simulink model "MATE_9LevelDrive_LowHarmonicRectifier"  (R2024b)
settings: Solver=FixedStepDiscrete  StartTime=0.0  StopTime=1  FixedStep=Ts  RelTol=1e-3
PostLoadFcn:
  | Ts=25e-6; initDrive9Level;Rsnu=30; Csnu=3e-6;Ron=0.01;Roff=1e6; Vf=2;
InitFcn:
  | Ts=25e-6; initDrive9Level;Rsnu=30; Csnu=3e-6;Ron=0.01;Roff=1e6; Vf=2;
values from neighbouring files (symbols this model uses):
  Lbase = Zbase/wbase    (= 0.0044902914611)    [initDrive9Level.m]
  Rgnd_rectifier = 1e4    (= 10000)    [initDrive9Level.m]
  T_2wind_ratio = 0.2677    [initDrive9Level.m]
  T_Lpu = Ltot_pu*9/10    (= 0.036)    [initDrive9Level.m]
  T_Lpu_pri = Ltot_pu/10    (= 0.004)    [initDrive9Level.m]
  T_Rpu = Rtot_pu*9/10    (= 0.009)    [initDrive9Level.m]
  T_Rpu_pri = Rtot_pu/10    (= 0.001)    [initDrive9Level.m]
  T_Vpri = 3000    [initDrive9Level.m]
  T_Vpri_15comp = 1.1168    [initDrive9Level.m]
  T_Vsec = 920    [initDrive9Level.m]
  Zbase = T_Vsec*T_Vsec/T_Pbase    (= 1.6928)    [initDrive9Level.m]
undefined symbols (not defined in the file or in its folder): DiscIntNeverNeededParam, gcbh, sps_rtmsupport
libraries: fl_lib x192, ee_lib x105, simetranss x26, nesl_utility x21
(part 5 of 5)

== system MATE_9LevelDrive_LowHarmonicRectifier/ModulationSimulink/Signal out ==
  freq(Hz) : Inport
  x : Inport  Port=2
  1pu-> 4 DC stage : Gain  Gain=4  SaturateOnIntegerOverflow=on  OutDataTypeStr=Inherit: Same as input  ParamDataTypeStr=Inherit: Same as input
  2*pi1 : Gain  Gain=2*pi  SaturateOnIntegerOverflow=on  OutDataTypeStr=Inherit: Same as input  ParamDataTypeStr=Inherit: Same as input
  Discrete-Time Integrator2 : DiscreteIntegrator  SampleTime=Ts  ICPrevOutput=DiscIntNeverNeededParam  ICPrevScaledInput=DiscIntNeverNeededParam
  Product : Product  SaturateOnIntegerOverflow=on  OutDataTypeStr=Inherit: Same as first input
  Sum : Sum  Inputs=|++  SaturateOnIntegerOverflow=on
  Trigonometric Function3 : Trigonometry
  phase : Constant  Value=[0 2*pi/3 -2*pi/3]
  Out1 : Outport  VectorParamsAs1DForOutWhenUnconnected=off
  wires:
  x/1 -> 1pu-> 4 DC stage/1
  Product/1 -> Out1/1
  1pu-> 4 DC stage/1 -> Product/2
  Trigonometric Function3/1 -> Product/1
  freq(Hz)/1 -> 2*pi1/1
  phase/1 -> Sum/2
  Sum/1 -> Trigonometric Function3/1
  Discrete-Time Integrator2/1 -> Sum/1
  2*pi1/1 -> Discrete-Time Integrator2/1

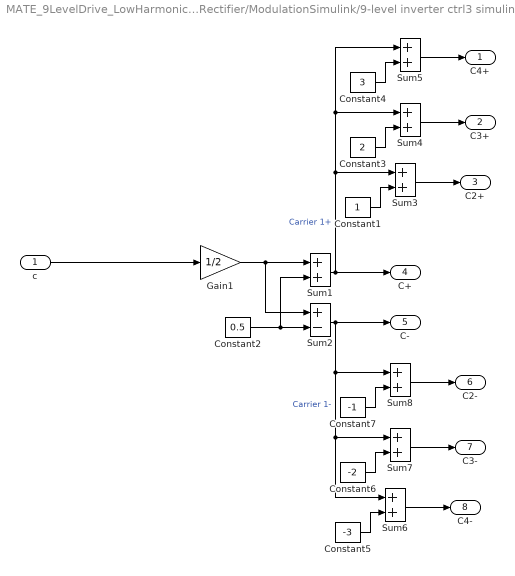
== system MATE_9LevelDrive_LowHarmonicRectifier/ModulationSimulink/9-level inverter ctrl3 simulink/Carriers Generator ==
  c : Inport
  Constant1 : Constant
  Constant2 : Constant  Value=0.5
  Constant3 : Constant  Value=2
  Constant4 : Constant  Value=3
  Constant5 : Constant  Value=-3
  Constant6 : Constant  Value=-2
  Constant7 : Constant  Value=-1
  Gain1 : Gain  Gain=1/2  SaturateOnIntegerOverflow=on  OutDataTypeStr=Inherit: Same as input  ParamDataTypeStr=Inherit: Same as input
  Sum{1,3..8} (7 alike) : Sum  InputSameDT=on  SaturateOnIntegerOverflow=on  OutDataTypeStr=Inherit: Same as first input
  Sum2 : Sum  Inputs=+-  InputSameDT=on  SaturateOnIntegerOverflow=on  OutDataTypeStr=Inherit: Same as first input
  C4+ : Outport  VectorParamsAs1DForOutWhenUnconnected=off
  C3+ : Outport  Port=2  VectorParamsAs1DForOutWhenUnconnected=off
  C2+ : Outport  Port=3  VectorParamsAs1DForOutWhenUnconnected=off
  C+ : Outport  Port=4  VectorParamsAs1DForOutWhenUnconnected=off
  C- : Outport  Port=5  VectorParamsAs1DForOutWhenUnconnected=off
  C2- : Outport  Port=6  VectorParamsAs1DForOutWhenUnconnected=off
  C3- : Outport  Port=7  VectorParamsAs1DForOutWhenUnconnected=off
  C4- : Outport  Port=8  VectorParamsAs1DForOutWhenUnconnected=off
  wires:
  c/1 -> Gain1/1
  Sum1/1 -> C+/1, Sum3/1, Sum4/1, Sum5/1  "Carrier 1+"
  Sum2/1 -> C-/1, Sum8/1, Sum7/1, Sum6/1  "Carrier 1-"
  Constant2/1 -> Sum1/2, Sum2/2
  Gain1/1 -> Sum2/1, Sum1/1
  Sum3/1 -> C2+/1
  Constant1/1 -> Sum3/2
  Sum4/1 -> C3+/1
  Constant3/1 -> Sum4/2
  Sum5/1 -> C4+/1
  Constant4/1 -> Sum5/2
  Sum6/1 -> C4-/1
  Constant5/1 -> Sum6/2
  Sum7/1 -> C3-/1
  Constant6/1 -> Sum7/2
  Sum8/1 -> C2-/1
  Constant7/1 -> Sum8/2

== system MATE_9LevelDrive_LowHarmonicRectifier/ModulationSimulink/9-level inverter ctrl3 simulink/rte1 ==
  in : Inport
  c+ : Inport  Port=2
  c- : Inport  Port=3
  Logical Operator : Logic  Operator=NOT  AllPortsSameDT=off  OutDataTypeStr=boolean
  Logical Operator1 : Logic  Operator=NOT  AllPortsSameDT=off  OutDataTypeStr=boolean
  Relational Operator : RelationalOperator  Operator=>  OutDataTypeStr=boolean  RndMeth=Simplest  InputSameDT=off
  Relational Operator1 : RelationalOperator  Operator=<  OutDataTypeStr=boolean  RndMeth=Simplest  InputSameDT=off
  1 : Outport  VectorParamsAs1DForOutWhenUnconnected=off
  2 : Outport  Port=2  VectorParamsAs1DForOutWhenUnconnected=off
  3 : Outport  Port=3  VectorParamsAs1DForOutWhenUnconnected=off
  4 : Outport  Port=4  VectorParamsAs1DForOutWhenUnconnected=off
  wires:
  Logical Operator1/1 -> 4/1
  Logical Operator/1 -> 2/1
  Relational Operator1/1 -> 3/1, Logical Operator1/1
  Relational Operator/1 -> 1/1, Logical Operator/1
  c-/1 -> Relational Operator1/2
  c+/1 -> Relational Operator/2
  in/1 -> Relational Operator/1, Relational Operator1/1

== system MATE_9LevelDrive_LowHarmonicRectifier/ModulationSimulink/9-level inverter ctrl3 simulink/rte2 ==
  in : Inport
  c+ : Inport  Port=2
  c- : Inport  Port=3
  Logical Operator : Logic  Operator=NOT  AllPortsSameDT=off  OutDataTypeStr=boolean
  Logical Operator1 : Logic  Operator=NOT  AllPortsSameDT=off  OutDataTypeStr=boolean
  Relational Operator : RelationalOperator  Operator=>  OutDataTypeStr=boolean  RndMeth=Simplest  InputSameDT=off
  Relational Operator1 : RelationalOperator  Operator=<  OutDataTypeStr=boolean  RndMeth=Simplest  InputSameDT=off
  1 : Outport  VectorParamsAs1DForOutWhenUnconnected=off
  2 : Outport  Port=2  VectorParamsAs1DForOutWhenUnconnected=off
  3 : Outport  Port=3  VectorParamsAs1DForOutWhenUnconnected=off
  4 : Outport  Port=4  VectorParamsAs1DForOutWhenUnconnected=off
  wires:
  in/1 -> Relational Operator1/1, Relational Operator/1
  c+/1 -> Relational Operator/2
  c-/1 -> Relational Operator1/2
  Relational Operator/1 -> Logical Operator/1, 1/1
  Relational Operator1/1 -> Logical Operator1/1, 3/1
  Logical Operator/1 -> 2/1
  Logical Operator1/1 -> 4/1

== system MATE_9LevelDrive_LowHarmonicRectifier/ModulationSimulink/9-level inverter ctrl3 simulink/rte3 ==
  in : Inport
  c+ : Inport  Port=2
  c- : Inport  Port=3
  Logical Operator : Logic  Operator=NOT  AllPortsSameDT=off  OutDataTypeStr=boolean
  Logical Operator1 : Logic  Operator=NOT  AllPortsSameDT=off  OutDataTypeStr=boolean
  Relational Operator : RelationalOperator  Operator=>  OutDataTypeStr=boolean  RndMeth=Simplest  InputSameDT=off
  Relational Operator1 : RelationalOperator  Operator=<  OutDataTypeStr=boolean  RndMeth=Simplest  InputSameDT=off
  1 : Outport  VectorParamsAs1DForOutWhenUnconnected=off
  2 : Outport  Port=2  VectorParamsAs1DForOutWhenUnconnected=off
  3 : Outport  Port=3  VectorParamsAs1DForOutWhenUnconnected=off
  4 : Outport  Port=4  VectorParamsAs1DForOutWhenUnconnected=off
  wires:
  in/1 -> Relational Operator1/1, Relational Operator/1
  c+/1 -> Relational Operator/2
  c-/1 -> Relational Operator1/2
  Relational Operator/1 -> Logical Operator/1, 1/1
  Relational Operator1/1 -> Logical Operator1/1, 3/1
  Logical Operator/1 -> 2/1
  Logical Operator1/1 -> 4/1

== system MATE_9LevelDrive_LowHarmonicRectifier/ModulationSimulink/9-level inverter ctrl3 simulink/rte4 ==
  in : Inport
  c+ : Inport  Port=2
  c- : Inport  Port=3
  Logical Operator : Logic  Operator=NOT  AllPortsSameDT=off  OutDataTypeStr=boolean
  Logical Operator1 : Logic  Operator=NOT  AllPortsSameDT=off  OutDataTypeStr=boolean
  Relational Operator : RelationalOperator  Operator=>  OutDataTypeStr=boolean  RndMeth=Simplest  InputSameDT=off
  Relational Operator1 : RelationalOperator  Operator=<  OutDataTypeStr=boolean  RndMeth=Simplest  InputSameDT=off
  1 : Outport  VectorParamsAs1DForOutWhenUnconnected=off
  2 : Outport  Port=2  VectorParamsAs1DForOutWhenUnconnected=off
  3 : Outport  Port=3  VectorParamsAs1DForOutWhenUnconnected=off
  4 : Outport  Port=4  VectorParamsAs1DForOutWhenUnconnected=off
  wires:
  Logical Operator1/1 -> 4/1
  Logical Operator/1 -> 2/1
  Relational Operator1/1 -> 3/1, Logical Operator1/1
  Relational Operator/1 -> 1/1, Logical Operator/1
  c-/1 -> Relational Operator1/2
  c+/1 -> Relational Operator/2
  in/1 -> Relational Operator/1, Relational Operator1/1

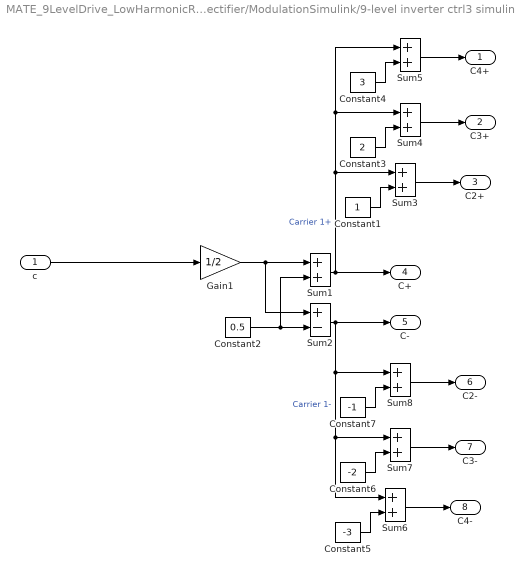
== system MATE_9LevelDrive_LowHarmonicRectifier/ModulationSimulink/9-level inverter ctrl3 simulink1/Carriers Generator ==
  c : Inport
  Constant1 : Constant
  Constant2 : Constant  Value=0.5
  Constant3 : Constant  Value=2
  Constant4 : Constant  Value=3
  Constant5 : Constant  Value=-3
  Constant6 : Constant  Value=-2
  Constant7 : Constant  Value=-1
  Gain1 : Gain  Gain=1/2  SaturateOnIntegerOverflow=on  OutDataTypeStr=Inherit: Same as input  ParamDataTypeStr=Inherit: Same as input
  Sum{1,3..8} (7 alike) : Sum  InputSameDT=on  SaturateOnIntegerOverflow=on  OutDataTypeStr=Inherit: Same as first input
  Sum2 : Sum  Inputs=+-  InputSameDT=on  SaturateOnIntegerOverflow=on  OutDataTypeStr=Inherit: Same as first input
  C4+ : Outport  VectorParamsAs1DForOutWhenUnconnected=off
  C3+ : Outport  Port=2  VectorParamsAs1DForOutWhenUnconnected=off
  C2+ : Outport  Port=3  VectorParamsAs1DForOutWhenUnconnected=off
  C+ : Outport  Port=4  VectorParamsAs1DForOutWhenUnconnected=off
  C- : Outport  Port=5  VectorParamsAs1DForOutWhenUnconnected=off
  C2- : Outport  Port=6  VectorParamsAs1DForOutWhenUnconnected=off
  C3- : Outport  Port=7  VectorParamsAs1DForOutWhenUnconnected=off
  C4- : Outport  Port=8  VectorParamsAs1DForOutWhenUnconnected=off
  wires:
  Constant7/1 -> Sum8/2
  Sum8/1 -> C2-/1
  Constant6/1 -> Sum7/2
  Sum7/1 -> C3-/1
  Constant5/1 -> Sum6/2
  Sum6/1 -> C4-/1
  Constant4/1 -> Sum5/2
  Sum5/1 -> C4+/1
  Constant3/1 -> Sum4/2
  Sum4/1 -> C3+/1
  Constant1/1 -> Sum3/2
  Sum3/1 -> C2+/1
  Gain1/1 -> Sum1/1, Sum2/1
  Constant2/1 -> Sum2/2, Sum1/2
  Sum2/1 -> Sum6/1, Sum7/1, Sum8/1, C-/1  "Carrier 1-"
  Sum1/1 -> Sum5/1, Sum4/1, Sum3/1, C+/1  "Carrier 1+"
  c/1 -> Gain1/1

== system MATE_9LevelDrive_LowHarmonicRectifier/ModulationSimulink/9-level inverter ctrl3 simulink1/rte1 ==
  in : Inport
  c+ : Inport  Port=2
  c- : Inport  Port=3
  Logical Operator : Logic  Operator=NOT  AllPortsSameDT=off  OutDataTypeStr=boolean
  Logical Operator1 : Logic  Operator=NOT  AllPortsSameDT=off  OutDataTypeStr=boolean
  Relational Operator : RelationalOperator  Operator=>  OutDataTypeStr=boolean  RndMeth=Simplest  InputSameDT=off
  Relational Operator1 : RelationalOperator  Operator=<  OutDataTypeStr=boolean  RndMeth=Simplest  InputSameDT=off
  1 : Outport  VectorParamsAs1DForOutWhenUnconnected=off
  2 : Outport  Port=2  VectorParamsAs1DForOutWhenUnconnected=off
  3 : Outport  Port=3  VectorParamsAs1DForOutWhenUnconnected=off
  4 : Outport  Port=4  VectorParamsAs1DForOutWhenUnconnected=off
  wires:
  in/1 -> Relational Operator1/1, Relational Operator/1
  c+/1 -> Relational Operator/2
  c-/1 -> Relational Operator1/2
  Relational Operator/1 -> Logical Operator/1, 1/1
  Relational Operator1/1 -> Logical Operator1/1, 3/1
  Logical Operator/1 -> 2/1
  Logical Operator1/1 -> 4/1

== system MATE_9LevelDrive_LowHarmonicRectifier/ModulationSimulink/9-level inverter ctrl3 simulink1/rte2 ==
  in : Inport
  c+ : Inport  Port=2
  c- : Inport  Port=3
  Logical Operator : Logic  Operator=NOT  AllPortsSameDT=off  OutDataTypeStr=boolean
  Logical Operator1 : Logic  Operator=NOT  AllPortsSameDT=off  OutDataTypeStr=boolean
  Relational Operator : RelationalOperator  Operator=>  OutDataTypeStr=boolean  RndMeth=Simplest  InputSameDT=off
  Relational Operator1 : RelationalOperator  Operator=<  OutDataTypeStr=boolean  RndMeth=Simplest  InputSameDT=off
  1 : Outport  VectorParamsAs1DForOutWhenUnconnected=off
  2 : Outport  Port=2  VectorParamsAs1DForOutWhenUnconnected=off
  3 : Outport  Port=3  VectorParamsAs1DForOutWhenUnconnected=off
  4 : Outport  Port=4  VectorParamsAs1DForOutWhenUnconnected=off
  wires:
  Logical Operator1/1 -> 4/1
  Logical Operator/1 -> 2/1
  Relational Operator1/1 -> 3/1, Logical Operator1/1
  Relational Operator/1 -> 1/1, Logical Operator/1
  c-/1 -> Relational Operator1/2
  c+/1 -> Relational Operator/2
  in/1 -> Relational Operator/1, Relational Operator1/1

== system MATE_9LevelDrive_LowHarmonicRectifier/ModulationSimulink/9-level inverter ctrl3 simulink1/rte3 ==
  in : Inport
  c+ : Inport  Port=2
  c- : Inport  Port=3
  Logical Operator : Logic  Operator=NOT  AllPortsSameDT=off  OutDataTypeStr=boolean
  Logical Operator1 : Logic  Operator=NOT  AllPortsSameDT=off  OutDataTypeStr=boolean
  Relational Operator : RelationalOperator  Operator=>  OutDataTypeStr=boolean  RndMeth=Simplest  InputSameDT=off
  Relational Operator1 : RelationalOperator  Operator=<  OutDataTypeStr=boolean  RndMeth=Simplest  InputSameDT=off
  1 : Outport  VectorParamsAs1DForOutWhenUnconnected=off
  2 : Outport  Port=2  VectorParamsAs1DForOutWhenUnconnected=off
  3 : Outport  Port=3  VectorParamsAs1DForOutWhenUnconnected=off
  4 : Outport  Port=4  VectorParamsAs1DForOutWhenUnconnected=off
  wires:
  Logical Operator1/1 -> 4/1
  Logical Operator/1 -> 2/1
  Relational Operator1/1 -> 3/1, Logical Operator1/1
  Relational Operator/1 -> 1/1, Logical Operator/1
  c-/1 -> Relational Operator1/2
  c+/1 -> Relational Operator/2
  in/1 -> Relational Operator/1, Relational Operator1/1

== system MATE_9LevelDrive_LowHarmonicRectifier/ModulationSimulink/9-level inverter ctrl3 simulink1/rte4 ==
  in : Inport
  c+ : Inport  Port=2
  c- : Inport  Port=3
  Logical Operator : Logic  Operator=NOT  AllPortsSameDT=off  OutDataTypeStr=boolean
  Logical Operator1 : Logic  Operator=NOT  AllPortsSameDT=off  OutDataTypeStr=boolean
  Relational Operator : RelationalOperator  Operator=>  OutDataTypeStr=boolean  RndMeth=Simplest  InputSameDT=off
  Relational Operator1 : RelationalOperator  Operator=<  OutDataTypeStr=boolean  RndMeth=Simplest  InputSameDT=off
  1 : Outport  VectorParamsAs1DForOutWhenUnconnected=off
  2 : Outport  Port=2  VectorParamsAs1DForOutWhenUnconnected=off
  3 : Outport  Port=3  VectorParamsAs1DForOutWhenUnconnected=off
  4 : Outport  Port=4  VectorParamsAs1DForOutWhenUnconnected=off
  wires:
  in/1 -> Relational Operator1/1, Relational Operator/1
  c+/1 -> Relational Operator/2
  c-/1 -> Relational Operator1/2
  Relational Operator/1 -> Logical Operator/1, 1/1
  Relational Operator1/1 -> Logical Operator1/1, 3/1
  Logical Operator/1 -> 2/1
  Logical Operator1/1 -> 4/1

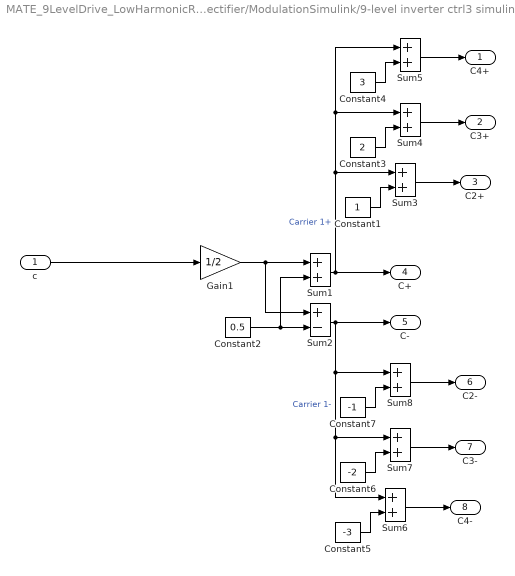
== system MATE_9LevelDrive_LowHarmonicRectifier/ModulationSimulink/9-level inverter ctrl3 simulink2/Carriers Generator ==
  c : Inport
  Constant1 : Constant
  Constant2 : Constant  Value=0.5
  Constant3 : Constant  Value=2
  Constant4 : Constant  Value=3
  Constant5 : Constant  Value=-3
  Constant6 : Constant  Value=-2
  Constant7 : Constant  Value=-1
  Gain1 : Gain  Gain=1/2  SaturateOnIntegerOverflow=on  OutDataTypeStr=Inherit: Same as input  ParamDataTypeStr=Inherit: Same as input
  Sum{1,3..8} (7 alike) : Sum  InputSameDT=on  SaturateOnIntegerOverflow=on  OutDataTypeStr=Inherit: Same as first input
  Sum2 : Sum  Inputs=+-  InputSameDT=on  SaturateOnIntegerOverflow=on  OutDataTypeStr=Inherit: Same as first input
  C4+ : Outport  VectorParamsAs1DForOutWhenUnconnected=off
  C3+ : Outport  Port=2  VectorParamsAs1DForOutWhenUnconnected=off
  C2+ : Outport  Port=3  VectorParamsAs1DForOutWhenUnconnected=off
  C+ : Outport  Port=4  VectorParamsAs1DForOutWhenUnconnected=off
  C- : Outport  Port=5  VectorParamsAs1DForOutWhenUnconnected=off
  C2- : Outport  Port=6  VectorParamsAs1DForOutWhenUnconnected=off
  C3- : Outport  Port=7  VectorParamsAs1DForOutWhenUnconnected=off
  C4- : Outport  Port=8  VectorParamsAs1DForOutWhenUnconnected=off
  wires:
  c/1 -> Gain1/1
  Sum1/1 -> C+/1, Sum3/1, Sum4/1, Sum5/1  "Carrier 1+"
  Sum2/1 -> C-/1, Sum8/1, Sum7/1, Sum6/1  "Carrier 1-"
  Constant2/1 -> Sum1/2, Sum2/2
  Gain1/1 -> Sum2/1, Sum1/1
  Sum3/1 -> C2+/1
  Constant1/1 -> Sum3/2
  Sum4/1 -> C3+/1
  Constant3/1 -> Sum4/2
  Sum5/1 -> C4+/1
  Constant4/1 -> Sum5/2
  Sum6/1 -> C4-/1
  Constant5/1 -> Sum6/2
  Sum7/1 -> C3-/1
  Constant6/1 -> Sum7/2
  Sum8/1 -> C2-/1
  Constant7/1 -> Sum8/2

== system MATE_9LevelDrive_LowHarmonicRectifier/ModulationSimulink/9-level inverter ctrl3 simulink2/rte1 ==
  in : Inport
  c+ : Inport  Port=2
  c- : Inport  Port=3
  Logical Operator : Logic  Operator=NOT  AllPortsSameDT=off  OutDataTypeStr=boolean
  Logical Operator1 : Logic  Operator=NOT  AllPortsSameDT=off  OutDataTypeStr=boolean
  Relational Operator : RelationalOperator  Operator=>  OutDataTypeStr=boolean  RndMeth=Simplest  InputSameDT=off
  Relational Operator1 : RelationalOperator  Operator=<  OutDataTypeStr=boolean  RndMeth=Simplest  InputSameDT=off
  1 : Outport  VectorParamsAs1DForOutWhenUnconnected=off
  2 : Outport  Port=2  VectorParamsAs1DForOutWhenUnconnected=off
  3 : Outport  Port=3  VectorParamsAs1DForOutWhenUnconnected=off
  4 : Outport  Port=4  VectorParamsAs1DForOutWhenUnconnected=off
  wires:
  Logical Operator1/1 -> 4/1
  Logical Operator/1 -> 2/1
  Relational Operator1/1 -> 3/1, Logical Operator1/1
  Relational Operator/1 -> 1/1, Logical Operator/1
  c-/1 -> Relational Operator1/2
  c+/1 -> Relational Operator/2
  in/1 -> Relational Operator/1, Relational Operator1/1

== system MATE_9LevelDrive_LowHarmonicRectifier/ModulationSimulink/9-level inverter ctrl3 simulink2/rte2 ==
  in : Inport
  c+ : Inport  Port=2
  c- : Inport  Port=3
  Logical Operator : Logic  Operator=NOT  AllPortsSameDT=off  OutDataTypeStr=boolean
  Logical Operator1 : Logic  Operator=NOT  AllPortsSameDT=off  OutDataTypeStr=boolean
  Relational Operator : RelationalOperator  Operator=>  OutDataTypeStr=boolean  RndMeth=Simplest  InputSameDT=off
  Relational Operator1 : RelationalOperator  Operator=<  OutDataTypeStr=boolean  RndMeth=Simplest  InputSameDT=off
  1 : Outport  VectorParamsAs1DForOutWhenUnconnected=off
  2 : Outport  Port=2  VectorParamsAs1DForOutWhenUnconnected=off
  3 : Outport  Port=3  VectorParamsAs1DForOutWhenUnconnected=off
  4 : Outport  Port=4  VectorParamsAs1DForOutWhenUnconnected=off
  wires:
  in/1 -> Relational Operator1/1, Relational Operator/1
  c+/1 -> Relational Operator/2
  c-/1 -> Relational Operator1/2
  Relational Operator/1 -> Logical Operator/1, 1/1
  Relational Operator1/1 -> Logical Operator1/1, 3/1
  Logical Operator/1 -> 2/1
  Logical Operator1/1 -> 4/1

== system MATE_9LevelDrive_LowHarmonicRectifier/ModulationSimulink/9-level inverter ctrl3 simulink2/rte3 ==
  in : Inport
  c+ : Inport  Port=2
  c- : Inport  Port=3
  Logical Operator : Logic  Operator=NOT  AllPortsSameDT=off  OutDataTypeStr=boolean
  Logical Operator1 : Logic  Operator=NOT  AllPortsSameDT=off  OutDataTypeStr=boolean
  Relational Operator : RelationalOperator  Operator=>  OutDataTypeStr=boolean  RndMeth=Simplest  InputSameDT=off
  Relational Operator1 : RelationalOperator  Operator=<  OutDataTypeStr=boolean  RndMeth=Simplest  InputSameDT=off
  1 : Outport  VectorParamsAs1DForOutWhenUnconnected=off
  2 : Outport  Port=2  VectorParamsAs1DForOutWhenUnconnected=off
  3 : Outport  Port=3  VectorParamsAs1DForOutWhenUnconnected=off
  4 : Outport  Port=4  VectorParamsAs1DForOutWhenUnconnected=off
  wires:
  in/1 -> Relational Operator1/1, Relational Operator/1
  c+/1 -> Relational Operator/2
  c-/1 -> Relational Operator1/2
  Relational Operator/1 -> Logical Operator/1, 1/1
  Relational Operator1/1 -> Logical Operator1/1, 3/1
  Logical Operator/1 -> 2/1
  Logical Operator1/1 -> 4/1

== system MATE_9LevelDrive_LowHarmonicRectifier/ModulationSimulink/9-level inverter ctrl3 simulink2/rte4 ==
  in : Inport
  c+ : Inport  Port=2
  c- : Inport  Port=3
  Logical Operator : Logic  Operator=NOT  AllPortsSameDT=off  OutDataTypeStr=boolean
  Logical Operator1 : Logic  Operator=NOT  AllPortsSameDT=off  OutDataTypeStr=boolean
  Relational Operator : RelationalOperator  Operator=>  OutDataTypeStr=boolean  RndMeth=Simplest  InputSameDT=off
  Relational Operator1 : RelationalOperator  Operator=<  OutDataTypeStr=boolean  RndMeth=Simplest  InputSameDT=off
  1 : Outport  VectorParamsAs1DForOutWhenUnconnected=off
  2 : Outport  Port=2  VectorParamsAs1DForOutWhenUnconnected=off
  3 : Outport  Port=3  VectorParamsAs1DForOutWhenUnconnected=off
  4 : Outport  Port=4  VectorParamsAs1DForOutWhenUnconnected=off
  wires:
  Logical Operator1/1 -> 4/1
  Logical Operator/1 -> 2/1
  Relational Operator1/1 -> 3/1, Logical Operator1/1
  Relational Operator/1 -> 1/1, Logical Operator/1
  c-/1 -> Relational Operator1/2
  c+/1 -> Relational Operator/2
  in/1 -> Relational Operator/1, Relational Operator1/1
